simulink model "PubIfDecisionTOS_MDL"  (R2020b)
settings: configuration reference "DspaceConfig" (kept outside this file)
PostLoadFcn:
  | if any(exist('dsrtsu_mdlpostloadfcn', 'file') ~= 0), dsrtsu_mdlpostloadfcn('Execute', bdroot); end
InitFcn:
  | , if any(exist('dsmpb_private', 'file') ~= 0), dsmpb_private('dsmpb_mdlclblib', 'Init', bdroot); end,
undefined symbols (not defined in the file or in its folder): C_TOS_ACCEgoRAxletoFbumplength_m, C_TOS_ACCTargetFront_Flag, C_TOS_AEBJAPedObjDxThre_Val, C_TOS_AEBJAPedObjDyThre_Val, C_TOS_AEBJATargetSize_Val, C_TOS_AEBJAVehObjDxThre_Val, C_TOS_AEBJAVehObjDyThre_Val, C_TOS_AEBJuncPedTargetSize_Val, C_TOS_AEBLatObjDxThre_Val, C_TOS_AEBLatPedDyThre_Val, C_TOS_AEBLatTargetSize_Val, C_TOS_AEBLongTargetInEgoFront_Flag, C_TOS_axAbsGround_Parameter, C_TOS_CameraConfirmedFlag, C_TOS_CNsubjWidth, C_TOS_CurrentLaneCoreMinWidth_Val, C_TOS_CutInProb_Val_Zero, C_TOS_CutOutProb_Val_Zero, C_TOS_D2R_Val, C_TOS_DefaultValueObjectToCenterLine_dy, C_TOS_EgoCarWidth_Val, C_TOS_EgoDxRefPoint_m, C_TOS_EgoRAxletoFbumplength_m, C_TOS_HalfWidthVehicle_Con, C_TOS_HWA_CurrentLaneFlag, C_TOS_HWA_LeftLaneFlag, C_TOS_HWA_MovingDir_Vaild, C_TOS_HWA_MovState_Vaild, C_TOS_HWA_RightLaneFlag, C_TOS_LaneLineCourseErrorFront, C_TOS_LaneLineCourseErrorRear, C_TOS_MotorbikeDefaultWidth_m, C_TOS_NumberOfEffectiveTargets, C_TOS_Obj_Age_Val, C_TOS_Objdx_Constraint_Val, C_TOS_ObjectDefaultWidth_m, C_TOS_ObjInCurrentLane_Val, C_TOS_ObjInCurrentLaneValid, C_TOS_ObjInLeftLaneValid, C_TOS_ObjInRightLaneValid, C_TOS_ObjNotInCurrentLane_Val, C_TOS_ObjNotREElementType, C_TOS_ObjPredictDis_dy_ConstantVal_Zeros, C_TOS_ObjToCenterLine_ConstantVal_Zeros, C_TOS_OFMObjIDInvilad_Val, C_TOS_PIL_LatDisCons_Val_zero, C_TOS_PIL_ObjectCutInFlag_b, C_TOS_PIL_ObjectCutOutFlag_b, C_TOS_PIL_ObjLaneProb_al_Val, C_TOS_PP_ObjFusType_FC_Confirm_b, C_TOS_PP_ObjFusType_FC_FR_Confirm_b, C_TOS_PP_ObjFusType_FR_Confirm_b, C_TOS_RE_80BoolDefault_Val, C_TOS_RE_80Single181Default_Val, C_TOS_RE_80Single255Default_Val, C_TOS_RE_80Uint8Default_Val, C_TOS_RE_D2R, C_TOS_RE_D_180_Val, C_TOS_RE_InvalidObjectID_Val, C_TOS_RE_InvalidTargetChainDir_Val ... (+142)
libraries: simulink x1650, TOS_LIB x361, canfdmsglib x14
(part 18 of 69)

== system PubIfDecisionTOS_MDL/TOS_20201112/TOS_2012080320/PP1128/ISV_InputSignalVerification/LM_SignalVerif/LM_RL_Bus/LM_RL_Line05 ==
  LM_Line05 : Inport
  Bus Creator2 : BusCreator  Inputs=8  OutDataTypeStr=Bus: TOS_LM_Line_bus  NonVirtualBus=on
      settings: InheritFromInputs=off
  Bus Selector2 : BusSelector  OutputSignals=pC0,pC1,pC2,pC3,dDisStart,dDisEnd,dQuality,fCamValid
  Signal Copy{1..7,24} (8 alike) : SignalConversion  OverrideOpt=off
  LM_RL_Line05 : Outport
  wires:
  Signal Copy1/1 -> Bus Creator2/2  "pC1"
  Bus Selector2/4 -> Signal Copy2/1  "<pC3>"
  Bus Creator2/1 -> LM_RL_Line05/1
  Signal Copy3/1 -> Bus Creator2/3  "pC2"
  Signal Copy6/1 -> Bus Creator2/5  "dDisStart"
  Signal Copy24/1 -> Bus Creator2/1  "pC0"
  Bus Selector2/1 -> Signal Copy24/1  "<pC0>"
  LM_Line05/1 -> Bus Selector2/1
  Bus Selector2/3 -> Signal Copy3/1  "<pC2>"
  Signal Copy4/1 -> Bus Creator2/6  "dDisEnd"
  Bus Selector2/5 -> Signal Copy6/1  "<dDisStart>"
  Bus Selector2/6 -> Signal Copy4/1  "<dDisEnd>"
  Bus Selector2/7 -> Signal Copy7/1  "<dQuality>"
  Bus Selector2/2 -> Signal Copy1/1  "<pC1>"
  Bus Selector2/8 -> Signal Copy5/1  "<fCamValid>"
  Signal Copy7/1 -> Bus Creator2/7  "dQuality"
  Signal Copy5/1 -> Bus Creator2/8  "fCamValid"
  Signal Copy2/1 -> Bus Creator2/4  "pC3"

== system PubIfDecisionTOS_MDL/TOS_20201112/TOS_2012080320/PP1128/ISV_InputSignalVerification/LM_SignalVerif/LM_RL_Bus/LM_RL_Line06 ==
  LM_Line06 : Inport
  Bus Creator2 : BusCreator  Inputs=8  OutDataTypeStr=Bus: TOS_LM_Line_bus  NonVirtualBus=on
      settings: InheritFromInputs=off
  Bus Selector2 : BusSelector  OutputSignals=pC0,pC1,pC2,pC3,dDisStart,dDisEnd,dQuality,fCamValid
  Signal Copy{1..7,24} (8 alike) : SignalConversion  OverrideOpt=off
  LM_RL_Line06 : Outport
  wires:
  Signal Copy2/1 -> Bus Creator2/4  "pC3"
  Signal Copy5/1 -> Bus Creator2/8  "fCamValid"
  Signal Copy7/1 -> Bus Creator2/7  "dQuality"
  Bus Selector2/8 -> Signal Copy5/1  "<fCamValid>"
  Bus Selector2/2 -> Signal Copy1/1  "<pC1>"
  Bus Selector2/7 -> Signal Copy7/1  "<dQuality>"
  Bus Selector2/6 -> Signal Copy4/1  "<dDisEnd>"
  Bus Selector2/5 -> Signal Copy6/1  "<dDisStart>"
  Signal Copy4/1 -> Bus Creator2/6  "dDisEnd"
  Bus Selector2/3 -> Signal Copy3/1  "<pC2>"
  LM_Line06/1 -> Bus Selector2/1
  Bus Selector2/1 -> Signal Copy24/1  "<pC0>"
  Signal Copy24/1 -> Bus Creator2/1  "pC0"
  Signal Copy6/1 -> Bus Creator2/5  "dDisStart"
  Signal Copy3/1 -> Bus Creator2/3  "pC2"
  Bus Creator2/1 -> LM_RL_Line06/1
  Bus Selector2/4 -> Signal Copy2/1  "<pC3>"
  Signal Copy1/1 -> Bus Creator2/2  "pC1"

== system PubIfDecisionTOS_MDL/TOS_20201112/TOS_2012080320/PP1128/ISV_InputSignalVerification/LM_SignalVerif/LM_RL_Bus/LM_RL_Line07 ==
  LM_Line07 : Inport
  Bus Creator2 : BusCreator  Inputs=8  OutDataTypeStr=Bus: TOS_LM_Line_bus  NonVirtualBus=on
      settings: InheritFromInputs=off
  Bus Selector2 : BusSelector  OutputSignals=pC0,pC1,pC2,pC3,dDisStart,dDisEnd,dQuality,fCamValid
  Signal Copy{1..7,24} (8 alike) : SignalConversion  OverrideOpt=off
  LM_RL_Line07 : Outport
  wires:
  Signal Copy1/1 -> Bus Creator2/2  "pC1"
  Bus Selector2/4 -> Signal Copy2/1  "<pC3>"
  Bus Creator2/1 -> LM_RL_Line07/1
  Signal Copy3/1 -> Bus Creator2/3  "pC2"
  Signal Copy6/1 -> Bus Creator2/5  "dDisStart"
  Signal Copy24/1 -> Bus Creator2/1  "pC0"
  Bus Selector2/1 -> Signal Copy24/1  "<pC0>"
  LM_Line07/1 -> Bus Selector2/1
  Bus Selector2/3 -> Signal Copy3/1  "<pC2>"
  Signal Copy4/1 -> Bus Creator2/6  "dDisEnd"
  Bus Selector2/5 -> Signal Copy6/1  "<dDisStart>"
  Bus Selector2/6 -> Signal Copy4/1  "<dDisEnd>"
  Bus Selector2/7 -> Signal Copy7/1  "<dQuality>"
  Bus Selector2/2 -> Signal Copy1/1  "<pC1>"
  Bus Selector2/8 -> Signal Copy5/1  "<fCamValid>"
  Signal Copy7/1 -> Bus Creator2/7  "dQuality"
  Signal Copy5/1 -> Bus Creator2/8  "fCamValid"
  Signal Copy2/1 -> Bus Creator2/4  "pC3"

== system PubIfDecisionTOS_MDL/TOS_20201112/TOS_2012080320/PP1128/ISV_InputSignalVerification/LM_SignalVerif/LM_RL_Bus/LM_RL_Line08 ==
  LM_Line08 : Inport
  Bus Creator2 : BusCreator  Inputs=8  OutDataTypeStr=Bus: TOS_LM_Line_bus  NonVirtualBus=on
      settings: InheritFromInputs=off
  Bus Selector2 : BusSelector  OutputSignals=pC0,pC1,pC2,pC3,dDisStart,dDisEnd,dQuality,fCamValid
  Signal Copy{1..7,24} (8 alike) : SignalConversion  OverrideOpt=off
  LM_RL_Line08 : Outport
  wires:
  Signal Copy2/1 -> Bus Creator2/4  "pC3"
  Signal Copy5/1 -> Bus Creator2/8  "fCamValid"
  Signal Copy7/1 -> Bus Creator2/7  "dQuality"
  Bus Selector2/8 -> Signal Copy5/1  "<fCamValid>"
  Bus Selector2/2 -> Signal Copy1/1  "<pC1>"
  Bus Selector2/7 -> Signal Copy7/1  "<dQuality>"
  Bus Selector2/6 -> Signal Copy4/1  "<dDisEnd>"
  Bus Selector2/5 -> Signal Copy6/1  "<dDisStart>"
  Signal Copy4/1 -> Bus Creator2/6  "dDisEnd"
  Bus Selector2/3 -> Signal Copy3/1  "<pC2>"
  LM_Line08/1 -> Bus Selector2/1
  Bus Selector2/1 -> Signal Copy24/1  "<pC0>"
  Signal Copy24/1 -> Bus Creator2/1  "pC0"
  Signal Copy6/1 -> Bus Creator2/5  "dDisStart"
  Signal Copy3/1 -> Bus Creator2/3  "pC2"
  Bus Creator2/1 -> LM_RL_Line08/1
  Bus Selector2/4 -> Signal Copy2/1  "<pC3>"
  Signal Copy1/1 -> Bus Creator2/2  "pC1"

== system PubIfDecisionTOS_MDL/TOS_20201112/TOS_2012080320/PP1128/ISV_InputSignalVerification/LM_SignalVerif/LM_RR_Bus/LM_RR_Line01 ==
  LM_Line01 : Inport
  Bus Creator2 : BusCreator  Inputs=8  OutDataTypeStr=Bus: TOS_LM_Line_bus  NonVirtualBus=on
      settings: InheritFromInputs=off
  Bus Selector2 : BusSelector  OutputSignals=pC0,pC1,pC2,pC3,dDisStart,dDisEnd,dQuality,fCamValid
  Signal Copy{1..7,24} (8 alike) : SignalConversion  OverrideOpt=off
  LM_RR_Line01 : Outport
  wires:
  Signal Copy2/1 -> Bus Creator2/4  "pC3"
  Signal Copy5/1 -> Bus Creator2/8  "fCamValid"
  Signal Copy7/1 -> Bus Creator2/7  "dQuality"
  Bus Selector2/8 -> Signal Copy5/1  "<fCamValid>"
  Bus Selector2/2 -> Signal Copy1/1  "<pC1>"
  Bus Selector2/7 -> Signal Copy7/1  "<dQuality>"
  Bus Selector2/6 -> Signal Copy4/1  "<dDisEnd>"
  Bus Selector2/5 -> Signal Copy6/1  "<dDisStart>"
  Signal Copy4/1 -> Bus Creator2/6  "dDisEnd"
  Bus Selector2/3 -> Signal Copy3/1  "<pC2>"
  LM_Line01/1 -> Bus Selector2/1
  Bus Selector2/1 -> Signal Copy24/1  "<pC0>"
  Signal Copy24/1 -> Bus Creator2/1  "pC0"
  Signal Copy6/1 -> Bus Creator2/5  "dDisStart"
  Signal Copy3/1 -> Bus Creator2/3  "pC2"
  Bus Creator2/1 -> LM_RR_Line01/1
  Bus Selector2/4 -> Signal Copy2/1  "<pC3>"
  Signal Copy1/1 -> Bus Creator2/2  "pC1"

== system PubIfDecisionTOS_MDL/TOS_20201112/TOS_2012080320/PP1128/ISV_InputSignalVerification/LM_SignalVerif/LM_RR_Bus/LM_RR_Line02 ==
  LM_Line02 : Inport
  Bus Creator2 : BusCreator  Inputs=8  OutDataTypeStr=Bus: TOS_LM_Line_bus  NonVirtualBus=on
      settings: InheritFromInputs=off
  Bus Selector2 : BusSelector  OutputSignals=pC0,pC1,pC2,pC3,dDisStart,dDisEnd,dQuality,fCamValid
  Signal Copy{1..7,24} (8 alike) : SignalConversion  OverrideOpt=off
  LM_RR_Line02 : Outport
  wires:
  Signal Copy1/1 -> Bus Creator2/2  "pC1"
  Bus Selector2/4 -> Signal Copy2/1  "<pC3>"
  Bus Creator2/1 -> LM_RR_Line02/1
  Signal Copy3/1 -> Bus Creator2/3  "pC2"
  Signal Copy6/1 -> Bus Creator2/5  "dDisStart"
  Signal Copy24/1 -> Bus Creator2/1  "pC0"
  Bus Selector2/1 -> Signal Copy24/1  "<pC0>"
  LM_Line02/1 -> Bus Selector2/1
  Bus Selector2/3 -> Signal Copy3/1  "<pC2>"
  Signal Copy4/1 -> Bus Creator2/6  "dDisEnd"
  Bus Selector2/5 -> Signal Copy6/1  "<dDisStart>"
  Bus Selector2/6 -> Signal Copy4/1  "<dDisEnd>"
  Bus Selector2/7 -> Signal Copy7/1  "<dQuality>"
  Bus Selector2/2 -> Signal Copy1/1  "<pC1>"
  Bus Selector2/8 -> Signal Copy5/1  "<fCamValid>"
  Signal Copy7/1 -> Bus Creator2/7  "dQuality"
  Signal Copy5/1 -> Bus Creator2/8  "fCamValid"
  Signal Copy2/1 -> Bus Creator2/4  "pC3"

== system PubIfDecisionTOS_MDL/TOS_20201112/TOS_2012080320/PP1128/ISV_InputSignalVerification/LM_SignalVerif/LM_RR_Bus/LM_RR_Line03 ==
  LM_Line03 : Inport
  Bus Creator2 : BusCreator  Inputs=8  OutDataTypeStr=Bus: TOS_LM_Line_bus  NonVirtualBus=on
      settings: InheritFromInputs=off
  Bus Selector2 : BusSelector  OutputSignals=pC0,pC1,pC2,pC3,dDisStart,dDisEnd,dQuality,fCamValid
  Signal Copy{1..7,24} (8 alike) : SignalConversion  OverrideOpt=off
  LM_RR_Line03 : Outport
  wires:
  Signal Copy2/1 -> Bus Creator2/4  "pC3"
  Signal Copy5/1 -> Bus Creator2/8  "fCamValid"
  Signal Copy7/1 -> Bus Creator2/7  "dQuality"
  Bus Selector2/8 -> Signal Copy5/1  "<fCamValid>"
  Bus Selector2/2 -> Signal Copy1/1  "<pC1>"
  Bus Selector2/7 -> Signal Copy7/1  "<dQuality>"
  Bus Selector2/6 -> Signal Copy4/1  "<dDisEnd>"
  Bus Selector2/5 -> Signal Copy6/1  "<dDisStart>"
  Signal Copy4/1 -> Bus Creator2/6  "dDisEnd"
  Bus Selector2/3 -> Signal Copy3/1  "<pC2>"
  LM_Line03/1 -> Bus Selector2/1
  Bus Selector2/1 -> Signal Copy24/1  "<pC0>"
  Signal Copy24/1 -> Bus Creator2/1  "pC0"
  Signal Copy6/1 -> Bus Creator2/5  "dDisStart"
  Signal Copy3/1 -> Bus Creator2/3  "pC2"
  Bus Creator2/1 -> LM_RR_Line03/1
  Bus Selector2/4 -> Signal Copy2/1  "<pC3>"
  Signal Copy1/1 -> Bus Creator2/2  "pC1"

== system PubIfDecisionTOS_MDL/TOS_20201112/TOS_2012080320/PP1128/ISV_InputSignalVerification/LM_SignalVerif/LM_RR_Bus/LM_RR_Line04 ==
  LM_Line04 : Inport
  Bus Creator2 : BusCreator  Inputs=8  OutDataTypeStr=Bus: TOS_LM_Line_bus  NonVirtualBus=on
      settings: InheritFromInputs=off
  Bus Selector2 : BusSelector  OutputSignals=pC0,pC1,pC2,pC3,dDisStart,dDisEnd,dQuality,fCamValid
  Signal Copy{1..7,24} (8 alike) : SignalConversion  OverrideOpt=off
  LM_RR_Line04 : Outport
  wires:
  Signal Copy1/1 -> Bus Creator2/2  "pC1"
  Bus Selector2/4 -> Signal Copy2/1  "<pC3>"
  Bus Creator2/1 -> LM_RR_Line04/1
  Signal Copy3/1 -> Bus Creator2/3  "pC2"
  Signal Copy6/1 -> Bus Creator2/5  "dDisStart"
  Signal Copy24/1 -> Bus Creator2/1  "pC0"
  Bus Selector2/1 -> Signal Copy24/1  "<pC0>"
  LM_Line04/1 -> Bus Selector2/1
  Bus Selector2/3 -> Signal Copy3/1  "<pC2>"
  Signal Copy4/1 -> Bus Creator2/6  "dDisEnd"
  Bus Selector2/5 -> Signal Copy6/1  "<dDisStart>"
  Bus Selector2/6 -> Signal Copy4/1  "<dDisEnd>"
  Bus Selector2/7 -> Signal Copy7/1  "<dQuality>"
  Bus Selector2/2 -> Signal Copy1/1  "<pC1>"
  Bus Selector2/8 -> Signal Copy5/1  "<fCamValid>"
  Signal Copy7/1 -> Bus Creator2/7  "dQuality"
  Signal Copy5/1 -> Bus Creator2/8  "fCamValid"
  Signal Copy2/1 -> Bus Creator2/4  "pC3"

== system PubIfDecisionTOS_MDL/TOS_20201112/TOS_2012080320/PP1128/ISV_InputSignalVerification/LM_SignalVerif/LM_RR_Bus/LM_RR_Line05 ==
  LM_Line05 : Inport
  Bus Creator2 : BusCreator  Inputs=8  OutDataTypeStr=Bus: TOS_LM_Line_bus  NonVirtualBus=on
      settings: InheritFromInputs=off
  Bus Selector2 : BusSelector  OutputSignals=pC0,pC1,pC2,pC3,dDisStart,dDisEnd,dQuality,fCamValid
  Signal Copy{1..7,24} (8 alike) : SignalConversion  OverrideOpt=off
  LM_RR_Line05 : Outport
  wires:
  Signal Copy2/1 -> Bus Creator2/4  "pC3"
  Signal Copy5/1 -> Bus Creator2/8  "fCamValid"
  Signal Copy7/1 -> Bus Creator2/7  "dQuality"
  Bus Selector2/8 -> Signal Copy5/1  "<fCamValid>"
  Bus Selector2/2 -> Signal Copy1/1  "<pC1>"
  Bus Selector2/7 -> Signal Copy7/1  "<dQuality>"
  Bus Selector2/6 -> Signal Copy4/1  "<dDisEnd>"
  Bus Selector2/5 -> Signal Copy6/1  "<dDisStart>"
  Signal Copy4/1 -> Bus Creator2/6  "dDisEnd"
  Bus Selector2/3 -> Signal Copy3/1  "<pC2>"
  LM_Line05/1 -> Bus Selector2/1
  Bus Selector2/1 -> Signal Copy24/1  "<pC0>"
  Signal Copy24/1 -> Bus Creator2/1  "pC0"
  Signal Copy6/1 -> Bus Creator2/5  "dDisStart"
  Signal Copy3/1 -> Bus Creator2/3  "pC2"
  Bus Creator2/1 -> LM_RR_Line05/1
  Bus Selector2/4 -> Signal Copy2/1  "<pC3>"
  Signal Copy1/1 -> Bus Creator2/2  "pC1"

== system PubIfDecisionTOS_MDL/TOS_20201112/TOS_2012080320/PP1128/ISV_InputSignalVerification/LM_SignalVerif/LM_RR_Bus/LM_RR_Line06 ==
  LM_Line06 : Inport
  Bus Creator2 : BusCreator  Inputs=8  OutDataTypeStr=Bus: TOS_LM_Line_bus  NonVirtualBus=on
      settings: InheritFromInputs=off
  Bus Selector2 : BusSelector  OutputSignals=pC0,pC1,pC2,pC3,dDisStart,dDisEnd,dQuality,fCamValid
  Signal Copy{1..7,24} (8 alike) : SignalConversion  OverrideOpt=off
  LM_RR_Line06 : Outport
  wires:
  Signal Copy1/1 -> Bus Creator2/2  "pC1"
  Bus Selector2/4 -> Signal Copy2/1  "<pC3>"
  Bus Creator2/1 -> LM_RR_Line06/1
  Signal Copy3/1 -> Bus Creator2/3  "pC2"
  Signal Copy6/1 -> Bus Creator2/5  "dDisStart"
  Signal Copy24/1 -> Bus Creator2/1  "pC0"
  Bus Selector2/1 -> Signal Copy24/1  "<pC0>"
  LM_Line06/1 -> Bus Selector2/1
  Bus Selector2/3 -> Signal Copy3/1  "<pC2>"
  Signal Copy4/1 -> Bus Creator2/6  "dDisEnd"
  Bus Selector2/5 -> Signal Copy6/1  "<dDisStart>"
  Bus Selector2/6 -> Signal Copy4/1  "<dDisEnd>"
  Bus Selector2/7 -> Signal Copy7/1  "<dQuality>"
  Bus Selector2/2 -> Signal Copy1/1  "<pC1>"
  Bus Selector2/8 -> Signal Copy5/1  "<fCamValid>"
  Signal Copy7/1 -> Bus Creator2/7  "dQuality"
  Signal Copy5/1 -> Bus Creator2/8  "fCamValid"
  Signal Copy2/1 -> Bus Creator2/4  "pC3"

== system PubIfDecisionTOS_MDL/TOS_20201112/TOS_2012080320/PP1128/ISV_InputSignalVerification/LM_SignalVerif/LM_RR_Bus/LM_RR_Line07 ==
  LM_Line07 : Inport
  Bus Creator2 : BusCreator  Inputs=8  OutDataTypeStr=Bus: TOS_LM_Line_bus  NonVirtualBus=on
      settings: InheritFromInputs=off
  Bus Selector2 : BusSelector  OutputSignals=pC0,pC1,pC2,pC3,dDisStart,dDisEnd,dQuality,fCamValid
  Signal Copy{1..7,24} (8 alike) : SignalConversion  OverrideOpt=off
  LM_RR_Line07 : Outport
  wires:
  Signal Copy2/1 -> Bus Creator2/4  "pC3"
  Signal Copy5/1 -> Bus Creator2/8  "fCamValid"
  Signal Copy7/1 -> Bus Creator2/7  "dQuality"
  Bus Selector2/8 -> Signal Copy5/1  "<fCamValid>"
  Bus Selector2/2 -> Signal Copy1/1  "<pC1>"
  Bus Selector2/7 -> Signal Copy7/1  "<dQuality>"
  Bus Selector2/6 -> Signal Copy4/1  "<dDisEnd>"
  Bus Selector2/5 -> Signal Copy6/1  "<dDisStart>"
  Signal Copy4/1 -> Bus Creator2/6  "dDisEnd"
  Bus Selector2/3 -> Signal Copy3/1  "<pC2>"
  LM_Line07/1 -> Bus Selector2/1
  Bus Selector2/1 -> Signal Copy24/1  "<pC0>"
  Signal Copy24/1 -> Bus Creator2/1  "pC0"
  Signal Copy6/1 -> Bus Creator2/5  "dDisStart"
  Signal Copy3/1 -> Bus Creator2/3  "pC2"
  Bus Creator2/1 -> LM_RR_Line07/1
  Bus Selector2/4 -> Signal Copy2/1  "<pC3>"
  Signal Copy1/1 -> Bus Creator2/2  "pC1"

== system PubIfDecisionTOS_MDL/TOS_20201112/TOS_2012080320/PP1128/ISV_InputSignalVerification/LM_SignalVerif/LM_RR_Bus/LM_RR_Line08 ==
  LM_Line08 : Inport
  Bus Creator2 : BusCreator  Inputs=8  OutDataTypeStr=Bus: TOS_LM_Line_bus  NonVirtualBus=on
      settings: InheritFromInputs=off
  Bus Selector2 : BusSelector  OutputSignals=pC0,pC1,pC2,pC3,dDisStart,dDisEnd,dQuality,fCamValid
  Signal Copy{1..7,24} (8 alike) : SignalConversion  OverrideOpt=off
  LM_RR_Line08 : Outport
  wires:
  Signal Copy1/1 -> Bus Creator2/2  "pC1"
  Bus Selector2/4 -> Signal Copy2/1  "<pC3>"
  Bus Creator2/1 -> LM_RR_Line08/1
  Signal Copy3/1 -> Bus Creator2/3  "pC2"
  Signal Copy6/1 -> Bus Creator2/5  "dDisStart"
  Signal Copy24/1 -> Bus Creator2/1  "pC0"
  Bus Selector2/1 -> Signal Copy24/1  "<pC0>"
  LM_Line08/1 -> Bus Selector2/1
  Bus Selector2/3 -> Signal Copy3/1  "<pC2>"
  Signal Copy4/1 -> Bus Creator2/6  "dDisEnd"
  Bus Selector2/5 -> Signal Copy6/1  "<dDisStart>"
  Bus Selector2/6 -> Signal Copy4/1  "<dDisEnd>"
  Bus Selector2/7 -> Signal Copy7/1  "<dQuality>"
  Bus Selector2/2 -> Signal Copy1/1  "<pC1>"
  Bus Selector2/8 -> Signal Copy5/1  "<fCamValid>"
  Signal Copy7/1 -> Bus Creator2/7  "dQuality"
  Signal Copy5/1 -> Bus Creator2/8  "fCamValid"
  Signal Copy2/1 -> Bus Creator2/4  "pC3"

== system PubIfDecisionTOS_MDL/TOS_20201112/TOS_2012080320/TLJ/Pro/Pro/ObjInLane/ObjInEgoLane_flag_1 ==
  Bus Creator : BusCreator  Inputs=4
  Constant1 : Constant  Value=0  OutDataTypeStr=boolean
  Constant2 : Constant  OutDataTypeStr=boolean
  Constant3 : Constant  Value=0  OutDataTypeStr=boolean
  Constant4 : Constant  OutDataTypeStr=uint8
  ObjInEgoLane_flag_1 : Outport
  wires:
  Constant3/1 -> Bus Creator/3  "ObjInRightLane_flag"
  Constant1/1 -> Bus Creator/1  "ObjInLeftLane_flag"
  Constant2/1 -> Bus Creator/2  "ObjInEgoLane_flag"
  Bus Creator/1 -> ObjInEgoLane_flag_1/1
  Constant4/1 -> Bus Creator/4  "TOS_TLJ_ObjInLaneCondition_Flag_ObserVale"

== system PubIfDecisionTOS_MDL/TOS_20201112/TOS_2012080320/TLJ/Pro/Pro/ObjInLane/ObjInEgoLane_flag_2 ==
  Bus Creator : BusCreator  Inputs=4
  Constant1 : Constant  Value=0  OutDataTypeStr=boolean
  Constant2 : Constant  OutDataTypeStr=boolean
  Constant3 : Constant  Value=0  OutDataTypeStr=boolean
  Constant4 : Constant  Value=4  OutDataTypeStr=uint8
  ObjInEgoLane_flag_1 : Outport
  wires:
  Bus Creator/1 -> ObjInEgoLane_flag_1/1
  Constant2/1 -> Bus Creator/2  "ObjInEgoLane_flag"
  Constant1/1 -> Bus Creator/1  "ObjInLeftLane_flag"
  Constant3/1 -> Bus Creator/3  "ObjInRightLane_flag"
  Constant4/1 -> Bus Creator/4  "TOS_TLJ_ObjInLaneCondition_Flag_ObserVale"

== system PubIfDecisionTOS_MDL/TOS_20201112/TOS_2012080320/TLJ/Pro/Pro/ObjInLane/ObjInEgoLane_flag_3 ==
  Bus Creator : BusCreator  Inputs=4
  Constant1 : Constant  Value=0  OutDataTypeStr=boolean
  Constant2 : Constant  OutDataTypeStr=boolean
  Constant3 : Constant  Value=0  OutDataTypeStr=boolean
  Constant4 : Constant  Value=5  OutDataTypeStr=uint8
  ObjInEgoLane_flag_1 : Outport
  wires:
  Constant3/1 -> Bus Creator/3  "ObjInRightLane_flag"
  Constant1/1 -> Bus Creator/1  "ObjInLeftLane_flag"
  Constant2/1 -> Bus Creator/2  "ObjInEgoLane_flag"
  Bus Creator/1 -> ObjInEgoLane_flag_1/1
  Constant4/1 -> Bus Creator/4  "TOS_TLJ_ObjInLaneCondition_Flag_ObserVale"

== system PubIfDecisionTOS_MDL/TOS_20201112/TOS_2012080320/TLJ/Pro/Pro/ObjInLane/ObjInLane_Default ==
  Bus Creator : BusCreator  Inputs=4
  Constant1 : Constant  Value=0  OutDataTypeStr=boolean
  Constant2 : Constant  Value=0  OutDataTypeStr=boolean
  Constant3 : Constant  Value=0  OutDataTypeStr=boolean
  Constant4 : Constant  Value=0  OutDataTypeStr=uint8
  ObjInEgoLane_flag_2 : Outport
  wires:
  Constant3/1 -> Bus Creator/3  "ObjInRightLane_flag"
  Constant1/1 -> Bus Creator/1  "ObjInLeftLane_flag"
  Constant2/1 -> Bus Creator/2  "ObjInEgoLane_flag"
  Bus Creator/1 -> ObjInEgoLane_flag_2/1
  Constant4/1 -> Bus Creator/4  "TOS_TLJ_ObjInLaneCondition_Flag_ObserVale"

== system PubIfDecisionTOS_MDL/TOS_20201112/TOS_2012080320/TLJ/Pro/Pro/ObjInLane/ObjInLeftLane_flag ==
  Bus Creator : BusCreator  Inputs=4
  Constant1 : Constant  OutDataTypeStr=boolean
  Constant2 : Constant  Value=0  OutDataTypeStr=boolean
  Constant3 : Constant  Value=0  OutDataTypeStr=boolean
  Constant4 : Constant  Value=2  OutDataTypeStr=uint8
  ObjInLeftLane_flag : Outport
  wires:
  Bus Creator/1 -> ObjInLeftLane_flag/1
  Constant2/1 -> Bus Creator/2  "ObjInEgoLane_flag"
  Constant1/1 -> Bus Creator/1  "ObjInLeftLane_flag"
  Constant3/1 -> Bus Creator/3  "ObjInRightLane_flag"
  Constant4/1 -> Bus Creator/4  "TOS_TLJ_ObjInLaneCondition_Flag_ObserVale"

== system PubIfDecisionTOS_MDL/TOS_20201112/TOS_2012080320/TLJ/Pro/Pro/ObjInLane/ObjInRightLane_flag ==
  Bus Creator : BusCreator  Inputs=4
  Constant1 : Constant  Value=0  OutDataTypeStr=boolean
  Constant2 : Constant  Value=0  OutDataTypeStr=boolean
  Constant3 : Constant  OutDataTypeStr=boolean
  Constant4 : Constant  Value=3  OutDataTypeStr=uint8
  ObjInRightLane_flag : Outport
  wires:
  Constant3/1 -> Bus Creator/3  "ObjInRightLane_flag"
  Constant1/1 -> Bus Creator/1  "ObjInLeftLane_flag"
  Constant2/1 -> Bus Creator/2  "ObjInEgoLane_flag"
  Bus Creator/1 -> ObjInRightLane_flag/1
  Constant4/1 -> Bus Creator/4  "TOS_TLJ_ObjInLaneCondition_Flag_ObserVale"

== system PubIfDecisionTOS_MDL/TOS_20201112/TOS_2012080320/TLJ/Pro/Pro/ObjInLane/TLJ_ObjInEgoLane_1 ==
  Object_Type : Inport
  TLJ_ObjinEgoLaneProb : Inport  Port=2
  "TLJ_ObjinLeftLaneProb " : Inport  Port=3
  "TLJ_ObjInRightlaneProb " : Inport  Port=4
  PIL_CutinFlag : Inport  Port=5
  PIL_CutoutFlag : Inport  Port=6
  Object_DY : Inport  Port=7
  Bus Creator : BusCreator  Inputs=7
  Bus Selector : BusSelector  OutputSignals=TLJ_ObjinEgoLaneProb,TLJ_ObjinLeftLaneProb
  Bus Selector1 : BusSelector  OutputSignals=TLJ_ObjinEgoLaneProb,TLJ_ObjInRightlaneProb
  Bus Selector2 : BusSelector  OutputSignals=TLJ_ObjinEgoLaneProb
  Bus Selector3 : BusSelector  OutputSignals=PIL_CutinFlag,PIL_CutoutFlag
  Compare To Constant1 : simulink/Logic and Bit Operations/Compare To Constant  relop===  const=C_TOS_PIL_ObjectCutInFlag_b  OutDataTypeStr=boolean
      settings: AttributesFormatString=C_TOS_PIL_ObjectCutInFlag_b = 1
  Compare To Constant2 : simulink/Logic and Bit Operations/Compare To Constant  relop=~=  const=C_TOS_PIL_ObjectCutOutFlag_b  OutDataTypeStr=boolean
      settings: AttributesFormatString=C_TOS_PIL_ObjectCutOutFlag_b = 1
  Compare To Constant5 : simulink/Logic and Bit Operations/Compare To Constant  relop=>  const=P_TOS_ObjinEgoLaneProb_Val  OutDataTypeStr=boolean
      settings: AttributesFormatString=P_TOS_ObjinEgoLaneProb_Val = 0.4
  Constant : Constant  OutDataTypeStr=boolean
  Logical Operator1 : Logic  Inputs=3  AllPortsSameDT=off  OutDataTypeStr=boolean
  Logical Operator2 : Logic  Operator=OR  AllPortsSameDT=off  OutDataTypeStr=boolean
  Logical Operator3 : Logic  AllPortsSameDT=off  OutDataTypeStr=boolean
  Prob : Subsystem  Commented=on
  Relational Operator : RelationalOperator  OutDataTypeStr=boolean  RndMeth=Nearest
  Relational Operator1 : RelationalOperator  OutDataTypeStr=boolean  RndMeth=Nearest
  Terminator : Terminator
  TLJ_ObjInEgoLane_flag : Outport
  wires:
  Logical Operator1/1 -> Logical Operator2/1
  Object_Type/1 -> Bus Creator/1  "Object_Type"
  PIL_CutinFlag/1 -> Bus Creator/5  "PIL_CutinFlag"
  "TLJ_ObjInRightlaneProb "/1 -> Bus Creator/4  "TLJ_ObjInRightlaneProb"
  "TLJ_ObjinLeftLaneProb "/1 -> Bus Creator/3  "TLJ_ObjinLeftLaneProb"
  TLJ_ObjinEgoLaneProb/1 -> Bus Creator/2  "TLJ_ObjinEgoLaneProb"
  Bus Creator/1 -> Bus Selector3/1, Bus Selector2/1, Bus Selector1/1, Bus Selector/1
  Bus Selector/1 -> Relational Operator/1  "<TLJ_ObjinEgoLaneProb>"
  Bus Selector/2 -> Relational Operator/2  "<TLJ_ObjinLeftLaneProb>"
  Bus Selector1/1 -> Relational Operator1/1  "<TLJ_ObjinEgoLaneProb>"
  Bus Selector1/2 -> Relational Operator1/2  "<TLJ_ObjInRightlaneProb>"
  Bus Selector2/1 -> Compare To Constant5/1  "<TLJ_ObjinEgoLaneProb>"
  Relational Operator1/1 -> Logical Operator1/2
  Relational Operator/1 -> Logical Operator1/1
  Compare To Constant5/1 -> Logical Operator1/3
  Object_DY/1 -> Bus Creator/7  "Object_DY"
  PIL_CutoutFlag/1 -> Bus Creator/6  "PIL_CutoutFlag"
  Bus Selector3/1 -> Compare To Constant1/1  "<PIL_CutinFlag>"
  Bus Selector3/2 -> Compare To Constant2/1  "<PIL_CutoutFlag>"
  Compare To Constant2/1 -> Terminator/1
  Compare To Constant1/1 -> Logical Operator2/2
  Logical Operator2/1 -> Logical Operator3/1
  Logical Operator3/1 -> TLJ_ObjInEgoLane_flag/1
  Constant/1 -> Logical Operator3/2

== system PubIfDecisionTOS_MDL/TOS_20201112/TOS_2012080320/TLJ/Pro/Pro/ObjInLane/TLJ_ObjInEgoLane_2 ==
  "PIL_ObjinEgoLaneProb " : Inport
  "PIL_ObjInLeftlaneProb " : Inport  Port=2
  "PIL_EgoVehicleInLeftlaneProb  " : Inport  Port=3
  "PIL_EgoVehicleInMiddlelaneProb  " : Inport  Port=4
  Compare To Constant1 : simulink/Logic and Bit Operations/Compare To Constant  relop=>  const=P_TOS_PIL_ObjInLeftlaneProb_Val  OutDataTypeStr=boolean
      settings: AttributesFormatString=P_TOS_PIL_ObjInLeftlaneProb_Val = 0.3
  Compare To Constant2 : simulink/Logic and Bit Operations/Compare To Constant  relop=>  const=P_TOS_PIL_EgoInLeftlaneProb_Val  OutDataTypeStr=boolean
      settings: AttributesFormatString=P_PIL_EgoInLeftlaneProb_Val = 0.3
  Compare To Constant3 : simulink/Logic and Bit Operations/Compare To Constant  relop=>  const=P_TOS_PIL_EgoInMiddlelaneProb_Val  OutDataTypeStr=boolean
      settings: AttributesFormatString=P_TOS_PIL_EgoInMiddlelaneProb_Val = 0.3
  Compare To Constant5 : simulink/Logic and Bit Operations/Compare To Constant  relop=>  const=P_TOS_PIL_ObjinEgoLaneProb_Val  OutDataTypeStr=boolean
      settings: AttributesFormatString=P_TOS_PIL_ObjinEgoLaneProb_Val = 0.3
  Logical Operator1 : Logic  Inputs=4  AllPortsSameDT=off  OutDataTypeStr=boolean
  TLJ_ObjInRightLane_flag : Outport
  wires:
  Logical Operator1/1 -> TLJ_ObjInRightLane_flag/1
  "PIL_ObjInLeftlaneProb "/1 -> Compare To Constant1/1
  "PIL_ObjinEgoLaneProb "/1 -> Compare To Constant5/1
  "PIL_EgoVehicleInLeftlaneProb  "/1 -> Compare To Constant2/1
  "PIL_EgoVehicleInMiddlelaneProb  "/1 -> Compare To Constant3/1
  Compare To Constant5/1 -> Logical Operator1/1
  Compare To Constant1/1 -> Logical Operator1/2
  Compare To Constant2/1 -> Logical Operator1/3
  Compare To Constant3/1 -> Logical Operator1/4

== system PubIfDecisionTOS_MDL/TOS_20201112/TOS_2012080320/TLJ/Pro/Pro/ObjInLane/TLJ_ObjInEgoLane_3 ==
  "PIL_ObjinEgoLaneProb " : Inport
  "PIL_ObjInRightlaneProb " : Inport  Port=2
  "PIL_EgoVehicleInRightlaneProb  " : Inport  Port=3
  "PIL_EgoVehicleInMiddlelaneProb  " : Inport  Port=4
  Compare To Constant1 : simulink/Logic and Bit Operations/Compare To Constant  relop=>  const=P_TOS_PIL_ObjInRightlaneProb_Val  OutDataTypeStr=boolean
      settings: AttributesFormatString=P_TOS_PIL_ObjInRightlaneProb_Val = 0.3
  Compare To Constant2 : simulink/Logic and Bit Operations/Compare To Constant  relop=>  const=P_TOS_PIL_EgoInRightlaneProb_Val  OutDataTypeStr=boolean
      settings: AttributesFormatString=P_TOS_PIL_EgoInRightlaneProb_Val = 0.3
  Compare To Constant7 : simulink/Logic and Bit Operations/Compare To Constant  relop=>  const=P_TOS_PIL_EgoInMiddlelaneProb_Val  OutDataTypeStr=boolean
      settings: AttributesFormatString=P_TOS_PIL_EgoInMiddlelaneProb_Val = 0.3
  Compare To Constant8 : simulink/Logic and Bit Operations/Compare To Constant  relop=>  const=P_TOS_PIL_ObjinEgoLaneProb_Val  OutDataTypeStr=boolean
      settings: AttributesFormatString=P_TOS_PIL_ObjinEgoLaneProb_Val = 0.3
  Logical Operator1 : Logic  Inputs=4  AllPortsSameDT=off  OutDataTypeStr=boolean
  TLJ_ObjInRightLane_flag : Outport
  wires:
  Compare To Constant7/1 -> Logical Operator1/4
  Compare To Constant2/1 -> Logical Operator1/3
  Compare To Constant1/1 -> Logical Operator1/2
  Compare To Constant8/1 -> Logical Operator1/1
  "PIL_EgoVehicleInMiddlelaneProb  "/1 -> Compare To Constant7/1
  "PIL_EgoVehicleInRightlaneProb  "/1 -> Compare To Constant2/1
  "PIL_ObjinEgoLaneProb "/1 -> Compare To Constant8/1
  "PIL_ObjInRightlaneProb "/1 -> Compare To Constant1/1
  Logical Operator1/1 -> TLJ_ObjInRightLane_flag/1

== system PubIfDecisionTOS_MDL/TOS_20201112/TOS_2012080320/TLJ/Pro/Pro/ObjInLane/TLJ_ObjInLeftLane ==
  TLJ_ObjinEgoLaneProb : Inport
  "TLJ_ObjinLeftLaneProb " : Inport  Port=2
  TLJ_ObjinRightLaneProb : Inport  Port=3
  Bus Creator : BusCreator  Inputs=3
  Bus Selector : BusSelector  OutputSignals=TLJ_ObjinLeftLaneProb,TLJ_ObjinEgoLaneProb
  Bus Selector1 : BusSelector  OutputSignals=TLJ_ObjinLeftLaneProb,TLJ_ObjinRightLaneProb
  Bus Selector2 : BusSelector  OutputSignals=TLJ_ObjinLeftLaneProb
  Compare To Constant5 : simulink/Logic and Bit Operations/Compare To Constant  relop=>  const=P_TOS_ObjinLeftLaneProb_Val  OutDataTypeStr=boolean
      settings: AttributesFormatString=P_TOS_ObjinLeftLaneProb_Val = 0.5
  Logical Operator1 : Logic  Inputs=3  AllPortsSameDT=off  OutDataTypeStr=boolean
  Relational Operator : RelationalOperator  Operator=>  OutDataTypeStr=boolean  RndMeth=Nearest
  Relational Operator1 : RelationalOperator  Operator=>  OutDataTypeStr=boolean  RndMeth=Nearest
  TLJ_ObjInLeftLane_flag : Outport
  wires:
  Compare To Constant5/1 -> Logical Operator1/3
  Relational Operator/1 -> Logical Operator1/1
  Relational Operator1/1 -> Logical Operator1/2
  Bus Selector2/1 -> Compare To Constant5/1  "<TLJ_ObjinLeftLaneProb>"
  Bus Selector1/2 -> Relational Operator1/2  "<TLJ_ObjinRightLaneProb>"
  Bus Selector1/1 -> Relational Operator1/1  "<TLJ_ObjinLeftLaneProb>"
  Bus Creator/1 -> Bus Selector/1, Bus Selector1/1, Bus Selector2/1
  TLJ_ObjinEgoLaneProb/1 -> Bus Creator/1  "TLJ_ObjinEgoLaneProb"
  "TLJ_ObjinLeftLaneProb "/1 -> Bus Creator/2  "TLJ_ObjinLeftLaneProb"
  TLJ_ObjinRightLaneProb/1 -> Bus Creator/3  "TLJ_ObjinRightLaneProb"
  Logical Operator1/1 -> TLJ_ObjInLeftLane_flag/1
  Bus Selector/1 -> Relational Operator/1  "<TLJ_ObjinLeftLaneProb>"
  Bus Selector/2 -> Relational Operator/2  "<TLJ_ObjinEgoLaneProb>"

== system PubIfDecisionTOS_MDL/TOS_20201112/TOS_2012080320/TLJ/Pro/Pro/ObjInLane/TLJ_ObjInRightLane ==
  TLJ_ObjinEgoLaneProb : Inport
  TLJ_ObjinLeftLaneProb : Inport  Port=2
  TLJ_ObjinRightLaneProb : Inport  Port=3
  Bus Creator : BusCreator  Inputs=3
  Bus Selector : BusSelector  OutputSignals=TLJ_ObjinRightLaneProb,TLJ_ObjinEgoLaneProb
  Bus Selector1 : BusSelector  OutputSignals=TLJ_ObjinRightLaneProb,TLJ_ObjinLeftLaneProb
  Bus Selector2 : BusSelector  OutputSignals=TLJ_ObjinRightLaneProb
  Compare To Constant5 : simulink/Logic and Bit Operations/Compare To Constant  relop=>  const=P_TOS_ObjinRightLaneProb_Val  OutDataTypeStr=boolean
      settings: AttributesFormatString=P_TOS_ObjinRightLaneProb_Val = 0.5
  Logical Operator1 : Logic  Inputs=3  AllPortsSameDT=off  OutDataTypeStr=boolean
  Relational Operator : RelationalOperator  Operator=>  OutDataTypeStr=boolean  RndMeth=Nearest
  Relational Operator1 : RelationalOperator  Operator=>  OutDataTypeStr=boolean  RndMeth=Nearest
  TLJ_ObjInRightLane_flag : Outport
  wires:
  Bus Selector/2 -> Relational Operator/2  "<TLJ_ObjinEgoLaneProb>"
  Bus Selector/1 -> Relational Operator/1  "<TLJ_ObjinRightLaneProb>"
  Logical Operator1/1 -> TLJ_ObjInRightLane_flag/1
  TLJ_ObjinRightLaneProb/1 -> Bus Creator/3  "TLJ_ObjinRightLaneProb"
  TLJ_ObjinLeftLaneProb/1 -> Bus Creator/2  "TLJ_ObjinLeftLaneProb"
  TLJ_ObjinEgoLaneProb/1 -> Bus Creator/1  "TLJ_ObjinEgoLaneProb"
  Bus Creator/1 -> Bus Selector2/1, Bus Selector1/1, Bus Selector/1
  Bus Selector2/1 -> Compare To Constant5/1  "<TLJ_ObjinRightLaneProb>"
  Relational Operator1/1 -> Logical Operator1/2
  Relational Operator/1 -> Logical Operator1/1
  Compare To Constant5/1 -> Logical Operator1/3
  Bus Selector1/1 -> Relational Operator1/1  "<TLJ_ObjinRightLaneProb>"
  Bus Selector1/2 -> Relational Operator1/2  "<TLJ_ObjinLeftLaneProb>"

== system PubIfDecisionTOS_MDL/TOS_20201112/TOS_2012080320/TOS/ACC/TOS_ACCCurrentLane/ACC_CurrentLane_Target/TOS_ACC_P0 ==
  ACC_P0_P1_Index : Inport
  Object_ID : Inport  Port=2
  Object_Fus_Type : Inport  Port=3
  object_MovingState : Inport  Port=4
  PP_ObjMovingDirSignalProcessing : Inport  Port=5
  Object_HeadingAngle : Inport  Port=6
  Object_DX : Inport  Port=7
  TOS_TLJ_SameLaneConfirm_Flag : Inport  Port=8
  Object_Type : Inport  Port=9
  Object_ObstacleProb : Inport  Port=10
  Object_DY : Inport  Port=11
  PP_ObjFusType_FC_FR_Confirm : Inport  Port=12
  PP_ObjFusType_FR_Confirm : Inport  Port=13
  PP_ObjFusType_FC_Confirm : Inport  Port=14
  Object_VX : Inport  Port=15
  Object_VY : Inport  Port=16
  VIE_EgoVelocity : Inport  Port=17
  SteerWheelAng : Inport  Port=18
  PIL_OverlapRatio : Inport  Port=19
  ACC_TargetP0_ID_K1 : Inport  Port=20
  ACC_TargetP0_ID_K2 : Inport  Port=21
  ACC_TargetP0_MovState_K1 : Inport  Port=22
  ACC_TargetP0_MovState_K2 : Inport  Port=23
  LM_LR_Line04_dDisStart : Inport  Port=24
  LM_LR_Line04_dDisEnd : Inport  Port=25
  LM_LR_Line05_dDisStart : Inport  Port=26
  LM_LR_Line05_dDisEnd : Inport  Port=27
  LM_LR_Line06_dDisStart : Inport  Port=28
  LM_LR_Line06_dDisEnd : Inport  Port=29
  LM_LR_Line04_pC2 : Inport  Port=30
  LM_LR_Line05_pC2 : Inport  Port=31
  LM_LR_Line06_pC2 : Inport  Port=32
  LM_LR_Line04_fCamValid : Inport  Port=33
  LM_LR_Line05_fCamValid : Inport  Port=34
  LM_LR_Line06_fCamValid : Inport  Port=35
  LM_LR_Line04_pC0 : Inport  Port=36
  LM_RL_Line04_pC0 : Inport  Port=37
  LM_LR_Line04_pC1 : Inport  Port=38
  LM_RL_Line04_pC1 : Inport  Port=39
  ACC_P0_Targe : Subsystem
  ACC_P0_TargeDefault : Subsystem  TreatAsAtomicUnit=on
  Compare To Constant : simulink/Logic and Bit Operations/Compare To Constant  relop===  const=C_TOS_OFMObjIDInvilad_Val  OutDataTypeStr=boolean
      settings: AttributesFormatString=C_TOS_OFMObjIDInvilad_Val = 0
  Constant1 : Constant  Value=0  OutDataTypeStr=uint8
  If : If  IfExpression=u1 ~= 0
  Merge{,1..18} (19 alike) : Merge
  Selector17 : Selector  InputPortWidth=2  IndexOptions=Index vector (dialog)  Indices=1  OutputSizes=1
  Switch1 : Switch  Criteria=u2 ~= 0
  TOS_ACC_P0_Index : Outport
  TOS_ACC_FusionType_ObserVale : Outport  Port=2
  TOS_ACC_TrgMovDir_ObserVale : Outport  Port=3
  TOS_ACC_TargetDxConfirm_ObserVale : Outport  Port=4
  TOS_ACC_ObjType_ObserVale : Outport  Port=5
  TOS_ACC_ObstacleProb_ObserVale : Outport  Port=6
  TOS_ACC_DyConfirm_ObserVale : Outport  Port=7
  TOS_ACC_TrgMovDirFlag_1_ObserVale : Outport  Port=8
  TOS_ACC_TrgMovDirFlag_2_ObserVale : Outport  Port=9
  TOS_ACC_TrgMovDirFlag_3_ObserVale : Outport  Port=10
  TOS_ACC_TrgMovDirFlag_4_ObserVale : Outport  Port=11
  TOS_ACC_TrgMovDirFlag_5_ObserVale : Outport  Port=12
  TOS_ACC_TrgMovDirFlag_6_ObserVale : Outport  Port=13
  TOS_ACC_DyConfirm_1_ObserVale : Outport  Port=14
  TOS_ACC_DyConfirm_2_ObserVale : Outport  Port=15
  TOS_ACC_DyConfirm_3_ObserVale : Outport  Port=16
  TOS_ACC_DyConfirm_4_OverlapRatio_ObserVale : Outport  Port=17
  TOS_ACC_DyConfirm_5_OverlapConfirm_ObserVale : Outport  Port=18
  TOS_ACC_DyConfirm_ALL_6_ObserVale : Outport  Port=19
  wires:
  If/1 -> ACC_P0_TargeDefault/Action
  Compare To Constant/1 -> If/1
  Merge1/1 -> TOS_ACC_FusionType_ObserVale/1
  Merge2/1 -> TOS_ACC_TrgMovDir_ObserVale/1
  Merge3/1 -> TOS_ACC_TargetDxConfirm_ObserVale/1
  Merge4/1 -> TOS_ACC_ObjType_ObserVale/1
  Merge5/1 -> TOS_ACC_ObstacleProb_ObserVale/1
  Merge6/1 -> TOS_ACC_DyConfirm_ObserVale/1
  [ACC_P0_Index] -> Switch1/1
  Merge/1 -> Switch1/2
  Constant1/1 -> Switch1/3
  ACC_P0_P1_Index/1 -> Selector17/1
  [ACC_P0_Index] -> ACC_P0_Targe/1(ACC_P0_Index)
  Object_Fus_Type/1 -> ACC_P0_Targe/2(Object_Fus_Type)
  object_MovingState/1 -> ACC_P0_Targe/3(object_MovingState)
  PP_ObjMovingDirSignalProcessing/1 -> ACC_P0_Targe/4(PP_ObjMovingDirSignalProcessing)
  Object_HeadingAngle/1 -> ACC_P0_Targe/5(Object_HeadingAngle)
  Object_DX/1 -> ACC_P0_Targe/6(Object_DX)
  TOS_TLJ_SameLaneConfirm_Flag/1 -> ACC_P0_Targe/7(TOS_TLJ_SameLaneConfirm_Flag)
  Object_Type/1 -> ACC_P0_Targe/8(Object_Type)
  Object_ObstacleProb/1 -> ACC_P0_Targe/9(Object_ObstacleProb)
  Object_DY/1 -> ACC_P0_Targe/10(Object_DY)
  ACC_P0_Targe/1(ACC_P0_TargeConfirm) -> Merge/2
  ACC_P0_Targe/2(TOS_ACC_FusionType_ObserVale) -> Merge1/2
  ACC_P0_Targe/3(TOS_ACC_TrgMovDir_ObserVale) -> Merge2/2
  ACC_P0_Targe/4(TOS_ACC_TargetDxConfirm_ObserVale) -> Merge3/2
  ACC_P0_Targe/5(TOS_ACC_ObjType_ObserVale) -> Merge4/2
  ACC_P0_Targe/6(TOS_ACC_ObstacleProb_ObserVale) -> Merge5/2
  ACC_P0_Targe/7(TOS_ACC_DyConfirm_ObserVale) -> Merge6/2
  If/2 -> ACC_P0_Targe/Action
  PP_ObjFusType_FC_Confirm/1 -> ACC_P0_Targe/13(PP_ObjFusType_FC_Confirm)
  PP_ObjFusType_FC_FR_Confirm/1 -> ACC_P0_Targe/11(PP_ObjFusType_FC_FR_Confirm)
  PP_ObjFusType_FR_Confirm/1 -> ACC_P0_Targe/12(PP_ObjFusType_FR_Confirm)
  Object_VY/1 -> ACC_P0_Targe/15(Object_VY)
  Object_VX/1 -> ACC_P0_Targe/14(Object_VX)
  VIE_EgoVelocity/1 -> ACC_P0_Targe/16(VIE_EgoVelocity)
  SteerWheelAng/1 -> ACC_P0_Targe/17(SteerWheelAng)
  PIL_OverlapRatio/1 -> ACC_P0_Targe/18(PIL_OverlapRatio)
  ACC_P0_Targe/8(TOS_ACC_TrgMovDirFlag_1_ObserVale) -> Merge7/2
  Merge7/1 -> TOS_ACC_TrgMovDirFlag_1_ObserVale/1
  ACC_TargetP0_ID_K1/1 -> ACC_P0_Targe/19(ACC_Target_ID_K1)
  ACC_TargetP0_ID_K2/1 -> ACC_P0_Targe/20(ACC_Target_ID_K2)
  ACC_TargetP0_MovState_K1/1 -> ACC_P0_Targe/21(ACC_Target_MovState_K1)
  ACC_TargetP0_MovState_K2/1 -> ACC_P0_Targe/22(ACC_Target_MovState_K2)
  Object_ID/1 -> ACC_P0_Targe/23(ObjectID)
  ACC_P0_Targe/13(TOS_ACC_TrgMovDirFlag_6_ObserVale) -> Merge8/2
  Merge8/1 -> TOS_ACC_TrgMovDirFlag_6_ObserVale/1
  Merge9/1 -> TOS_ACC_TrgMovDirFlag_2_ObserVale/1
  Merge10/1 -> TOS_ACC_TrgMovDirFlag_3_ObserVale/1
  Merge11/1 -> TOS_ACC_TrgMovDirFlag_4_ObserVale/1
  Merge12/1 -> TOS_ACC_TrgMovDirFlag_5_ObserVale/1
  ACC_P0_Targe/9(TOS_ACC_TrgMovDirFlag_2_ObserVale) -> Merge9/2
  ACC_P0_Targe/10(TOS_ACC_TrgMovDirFlag_3_ObserVale) -> Merge10/2
  ACC_P0_Targe/11(TOS_ACC_TrgMovDirFlag_4_ObserVale) -> Merge11/2
  ACC_P0_Targe/12(TOS_ACC_TrgMovDirFlag_5_ObserVale) -> Merge12/2
  ACC_P0_Targe/15(TOS_ACC_DyConfirm_2_ObserVale) -> Merge13/2
  ACC_P0_Targe/16(TOS_ACC_DyConfirm_3_ObserVale) -> Merge14/2
  ACC_P0_Targe/17(TOS_ACC_DyConfirm_4_OverlapRatio_ObserVale) -> Merge15/2
  Merge13/1 -> TOS_ACC_DyConfirm_2_ObserVale/1
  Merge14/1 -> TOS_ACC_DyConfirm_3_ObserVale/1
  Merge15/1 -> TOS_ACC_DyConfirm_4_OverlapRatio_ObserVale/1
  Selector17/1 -> [ACC_P0_Index], Compare To Constant/1
  Switch1/1 -> TOS_ACC_P0_Index/1
  Merge16/1 -> TOS_ACC_DyConfirm_1_ObserVale/1
  ACC_P0_Targe/14(TOS_ACC_DyConfirm_1_ObserVale) -> Merge16/2
  LM_LR_Line04_dDisStart/1 -> ACC_P0_Targe/24(LM_LR_Line04_dDisStart)
  LM_LR_Line04_dDisEnd/1 -> ACC_P0_Targe/25(LM_LR_Line04_dDisEnd)
  LM_LR_Line05_dDisStart/1 -> ACC_P0_Targe/26(LM_LR_Line05_dDisStart)
  LM_LR_Line05_dDisEnd/1 -> ACC_P0_Targe/27(LM_LR_Line05_dDisEnd)
  LM_LR_Line06_dDisStart/1 -> ACC_P0_Targe/28(LM_LR_Line06_dDisStart)
  LM_LR_Line06_dDisEnd/1 -> ACC_P0_Targe/29(LM_LR_Line06_dDisEnd)
  LM_LR_Line04_pC2/1 -> ACC_P0_Targe/30(LM_LR_Line04_pC2)
  LM_LR_Line05_pC2/1 -> ACC_P0_Targe/31(LM_LR_Line05_pC2)
  LM_LR_Line06_pC2/1 -> ACC_P0_Targe/32(LM_LR_Line06_pC2)
  LM_LR_Line04_fCamValid/1 -> ACC_P0_Targe/33(LM_LR_Line04_fCamValid)
  LM_LR_Line05_fCamValid/1 -> ACC_P0_Targe/34(LM_LR_Line05_fCamValid)
  LM_LR_Line06_fCamValid/1 -> ACC_P0_Targe/35(LM_LR_Line06_fCamValid)
  Merge17/1 -> TOS_ACC_DyConfirm_5_OverlapConfirm_ObserVale/1
  ACC_P0_Targe/18(TOS_ACC_DyConfirm_5_OverlapConfirm_ObserVale) -> Merge17/2
  ACC_P0_TargeDefault/1(ACC_P0_TargeConfirm) -> Merge/1
  ACC_P0_TargeDefault/2(TOS_ACC_FusionType_ObserVale) -> Merge1/1
  ACC_P0_TargeDefault/3(TOS_ACC_TrgMovDir_ObserVale) -> Merge2/1
  ACC_P0_TargeDefault/4(TOS_ACC_TargetDxConfirm_ObserVale) -> Merge3/1
  ACC_P0_TargeDefault/5(TOS_ACC_ObjType_ObserVale) -> Merge4/1
  ACC_P0_TargeDefault/6(TOS_ACC_ObstacleProb_ObserVale) -> Merge5/1
  ACC_P0_TargeDefault/7(TOS_ACC_DyConfirm_ObserVale) -> Merge6/1
  ACC_P0_TargeDefault/8(TOS_ACC_TrgMovDirFlag_1_ObserVale) -> Merge7/1
  ACC_P0_TargeDefault/9(TOS_ACC_TrgMovDirFlag_2_ObserVale) -> Merge9/1
  ACC_P0_TargeDefault/10(TOS_ACC_TrgMovDirFlag_3_ObserVale) -> Merge10/1
  ACC_P0_TargeDefault/11(TOS_ACC_TrgMovDirFlag_4_ObserVale) -> Merge11/1
  ACC_P0_TargeDefault/12(TOS_ACC_TrgMovDirFlag_5_ObserVale) -> Merge12/1
  ACC_P0_TargeDefault/13(TOS_ACC_TrgMovDirFlag_6_ObserVale) -> Merge8/1
  ACC_P0_TargeDefault/14(TOS_ACC_DyConfirm_1_ObserVale) -> Merge16/1
  ACC_P0_TargeDefault/15(TOS_ACC_DyConfirm_2_ObserVale) -> Merge13/1
  ACC_P0_TargeDefault/16(TOS_ACC_DyConfirm_3_ObserVale) -> Merge14/1
  ACC_P0_TargeDefault/17(TOS_ACC_DyConfirm_4_OverlapRatio_ObserVale) -> Merge15/1
  ACC_P0_TargeDefault/18(TOS_ACC_DyConfirm_5_OverlapConfirm_ObserVale) -> Merge17/1
  ACC_P0_Targe/19(TOS_ACC_DyConfirm_ALL_6_ObserVale) -> Merge18/2
  Merge18/1 -> TOS_ACC_DyConfirm_ALL_6_ObserVale/1
  ACC_P0_TargeDefault/19(TOS_ACC_DyConfirm_ALL_6_ObserVale1) -> Merge18/1
  LM_LR_Line04_pC0/1 -> ACC_P0_Targe/36(LM_LR_Line04_pC0)  "LM_LR_Line04_pC0"
  LM_RL_Line04_pC0/1 -> ACC_P0_Targe/37(LM_RL_Line04_pC0)  "LM_RL_Line04_pC0"
  LM_LR_Line04_pC1/1 -> ACC_P0_Targe/38(LM_LR_Line04_pC1)
  LM_RL_Line04_pC1/1 -> ACC_P0_Targe/39(LM_RL_Line04_pC1)
